simulink model "LTI"  (R2022a)
settings: Solver=VariableStepAuto  StartTime=0.0  StopTime=10.0  RelTol=1e-3
settings Model: Creator=Userx  LastModifiedBy=Userx

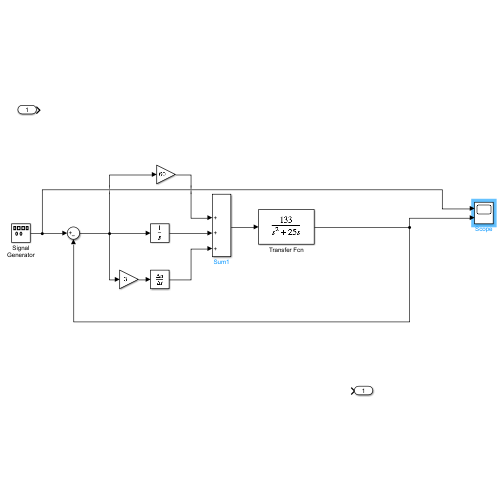
[thumbnail: Simulink's stored preview of the top-level diagram]
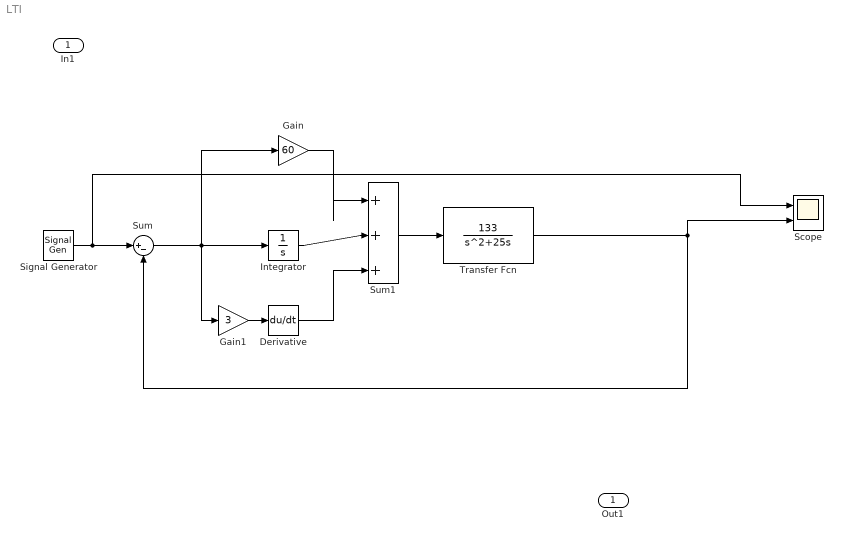
== system LTI ==
  In1 : Inport
  Derivative : Derivative
  Gain : Gain  Gain=60
  Gain1 : Gain  Gain=3
  Integrator : Integrator
  Scope : Scope  NumInputPorts=2
  Signal Generator : SignalGenerator  Frequency=0.4*pi  Units=rad/sec
  Sum : Sum  Inputs=|+-
  Sum1 : Sum  Inputs=|+++
  Transfer Fcn : TransferFcn  Numerator=[133]  Denominator=[1 25 0]
  Out1 : Outport
  wires:
  Signal Generator/1 -> Scope/1, Sum/1
  Sum/1 -> Gain1/1, Integrator/1, Gain/1
  Gain/1 -> Sum1/1
  Integrator/1 -> Sum1/2
  Derivative/1 -> Sum1/3
  Sum1/1 -> Transfer Fcn/1
  Transfer Fcn/1 -> Scope/2, Sum/2
  Gain1/1 -> Derivative/1
